simulink model "lorenz_sim"  (Simulink 6.3)
settings: Solver=ode4  StartTime=0.0  StopTime=5  FixedStep=0.01  RelTol=1e-3
undefined symbols (not defined in the file): b, delt, r, x0, y0, z0
settings Model: ModifiedByFormat=zhl_chosenone  LastModifiedBy=zhl_chosenone

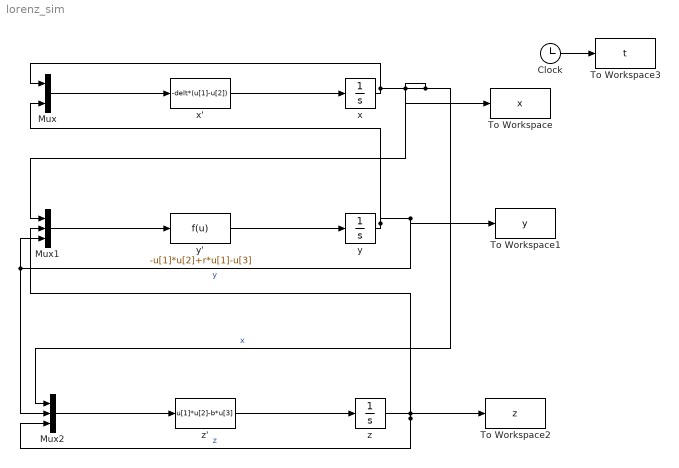
== system lorenz_sim ==
  Clock : Clock
      settings: Decimation=10
  Mux : Mux  Inputs=2
  Mux1 : Mux  Inputs=3
  Mux2 : Mux  Inputs=3
  To Workspace : ToWorkspace  VariableName=x  SampleTime=-1  SaveFormat=Array
  To Workspace1 : ToWorkspace  VariableName=y  SampleTime=-1  SaveFormat=Array
  To Workspace2 : ToWorkspace  VariableName=z  SampleTime=-1  SaveFormat=Array
  To Workspace3 : ToWorkspace  VariableName=t  SampleTime=-1  SaveFormat=Array
  x : Integrator  InitialCondition=x0
  x' : Fcn  Expr=-delt*(u[1]-u[2])
  y : Integrator  InitialCondition=y0
  y' : Fcn  Expr=-u[1]*u[2]+r*u[1]-u[3]
  z : Integrator  InitialCondition=z0
  z' : Fcn  Expr=u[1]*u[2]-b*u[3]
  wires:
  Mux/1 -> x'/1
  x'/1 -> x/1
  Mux1/1 -> y'/1
  y'/1 -> y/1
  Mux2/1 -> z'/1
  z'/1 -> z/1
  x/1 -> Mux/1, Mux1/1, Mux2/1, To Workspace/1  "x"
  y/1 -> Mux/2, Mux1/3, Mux2/2, To Workspace1/1  "y"
  z/1 -> Mux1/2, Mux2/3, To Workspace2/1  "z"
  Clock/1 -> To Workspace3/1
